simulink model "questao2MiguelSimItem4"  (Simulink 8.7)
settings: Solver=ode45  StartTime=0.0  StopTime=30  MaxStep=0.01  RelTol=1e-3
values from neighbouring files (symbols this model uses):
  A = [0 1  0              0 ... (first row only)    [MatLab4p.m]    (also in MatLab5p.m = [     0        1       0        0; MatLab6p_solucao4.m = [     0        1       0        0; MatLab7p.m = [0 1; -5*sqrt(2) -1]; pplane8.m = [)
  Am = blkdiag(M,M)    [MatLab5p.m]    (also in MatLab6p_solucao4.m; questao2Miguel.m = blkdiag(M); questao2MiguelFinal.m = blkdiag(M))
  Am2 = blkdiag(M)    [questao2Miguel.m]    (also in questao2MiguelFinal.m)
  B = [0; 1/M; 0; -1/(M*L)]    [MatLab4p.m]    (also in MatLab5p.m = [ 0    0; MatLab6p_solucao4.m = [ 0    0; MatLab7p.m = [0 ; 10]; pplane8.m = real(A))
  Bm = blkdiag(N,N)    [MatLab5p.m]    (also in MatLab6p_solucao4.m; questao2Miguel.m = blkdiag(N); questao2MiguelFinal.m = blkdiag(N))
  Bm2 = blkdiag(N)    [questao2Miguel.m]    (also in questao2MiguelFinal.m)
  C = [1 0 0 0]    [MatLab4p.m]    (also in MatLab5p.m = [1 0 0 0; MatLab6p_solucao4.m = [1 0 0 0; MatLab7p.m = [1 0]; pplane8.m = imag(A))
  Dsim = zeros(4,1)    [MatLab4p.m]    (also in MatLab5p.m = zeros(4,2); MatLab6p_solucao4.m = zeros(4,2); questao2Miguel.m; questao2MiguelFinal.m)
  g = 9.81    [MatLab4p.m]    (also in PenduloInvertidoNLinear.m; questao2Miguel.m; questao2MiguelFinal.m)
  K = place(A,B,[-3 -3.05 -3.1 -3.15])    [MatLab4p.m]    (also in MatLab5p.m = Ka(:,1:4); MatLab6p_solucao4.m = Ka(:,1:4); MatLab7p.m = place(A,B,[-4 -4.05]); pplane8.m = kk +2*(jj-1))
  K2 = Ka2(1:4)    [questao2Miguel.m]    (also in questao2MiguelFinal.m)
  Km = Ka(:,5:10)    [MatLab5p.m]    (also in MatLab6p_solucao4.m = Ka(:,5:12); MatLab7p.m = Ka(1,3); questao2Miguel.m = Ka(5); questao2MiguelFinal.m = Ka(5))
  Km2 = Ka2(5:6)    [questao2Miguel.m]    (also in questao2MiguelFinal.m)
  L = (place(A',C',[-9 -9.05 -9.1 -9.15]))'    [MatLab4p.m]    (also in MatLab7p.m = [23 ; 113.9289]; PenduloInvertidoNLinear.m = 1; pplane8.m = length(t); questao2Miguel.m = 1)
  Lobs = H'    [MatLab6p_solucao4.m]    (also in questao2Miguel.m; questao2MiguelFinal.m)
  m = 0.5    [MatLab4p.m]    (also in PenduloInvertidoNLinear.m; questao2Miguel.m; questao2MiguelFinal.m)
  Mcar = 1    [questao2MiguelFinal.m]
  x0 = [0 0 pi/4 0]    [MatLab4p.m]    (also in MatLab5p.m = [1 0.5 1 0.1]; MatLab6p_solucao4.m = [0 0 0 0]; MatLab7p.m = [0 ; 0]; questao2Miguel.m = [0 0.01 0.3 0])
  x0obs = [0 0 0 0]    [MatLab4p.m]    (also in MatLab6p_solucao4.m; MatLab7p.m = [0 ; 0]; questao2Miguel.m; questao2MiguelFinal.m)
settings Model: Creator=hector  LastModifiedBy=Deinis-UFSC
settings DebuggingCC: UnderspecifiedInitializationDetection=Simplified  MergeDetectMultiDrivingBlocksExec=error  SolverPrmCheckMsg=warning
settings ConfigComp: CovSFcnEnable=off

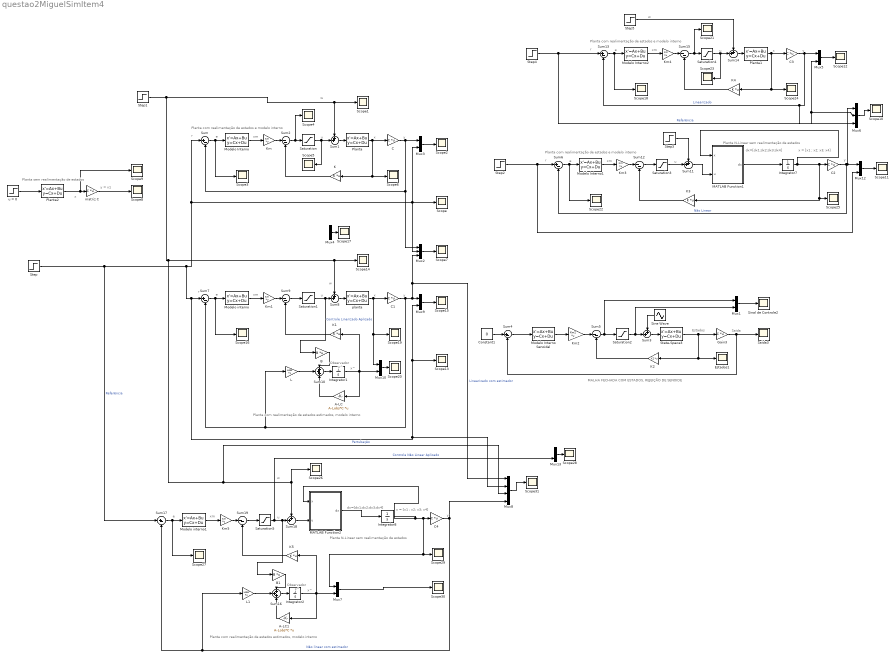
== system questao2MiguelSimItem4 ==
  note: Planta com realimentação de estados estimados, modelo interno
  note: Planta com realimentação de estados e modelo interno
  note: w
  note: u
  note: xm
  note: e
  note: r
  note: x
  note: y
  note: w
  note: u
  note: xm
  note: e
  note: r
  note: x
  note: y
  note: Observador
  note: x^
  note: x^
  note: Planta sem realimentação de estados
  note: x
  note: y = x1
  note: MALHA FECHADA COM ESTADOS, REJEIÇÃO DE SENOIDE
  note: Saida
  note: Estados
  note: Planta com realimentação de estados e modelo interno
  note: u
  note: xm
  note: e
  note: r
  note: y
  note: Planta N-Linear sem realimentação de estados
  note: dx=[dx1;dx2;dx3;dx4]
  note: x = [x1 ; x2; x3; x4]
  note: Planta com realimentação de estados e modelo interno
  note: w
  note: u
  note: xm
  note: e
  note: r
  note: x
  note: y
  note: Planta com realimentação de estados estimados, modelo interno
  note: w
  note: u
  note: xm
  note: e
  note: y
  note: Observador
  note: x^
  note: x^
  note: Planta N-Linear sem realimentação de estados
  note: dx=[dx1;dx2;dx3;dx4]
  note: x = [x1 ; x2; x3; x4]
  A-LC : Gain  Gain=A-Lobs*C  Multiplication=Matrix(K*u)
  A-LC1 : Gain  Gain=A-Lobs*C  Multiplication=Matrix(K*u)
  B : Gain  Gain=B  Multiplication=Matrix(K*u)
  B1 : Gain  Gain=B  Multiplication=Matrix(K*u)
  C{,1..4} (5 alike) : Gain  Gain=C  Multiplication=Matrix(K*u)
  Constant1 : Constant  Value=0
  Estados1 : Scope
  Gain3 : Gain  Gain=C  Multiplication=Matrix(K*u)
  Integrator1 : Integrator  InitialCondition=x0obs
  Integrator2 : Integrator  InitialCondition=x0obs
  Integrator7 : Integrator  InitialCondition=x0
  Integrator8 : Integrator  InitialCondition=x0
  K{,1,3..5} (5 alike) : Gain  Gain=K  Multiplication=Matrix(K*u)
  K2 : Gain  Gain=K2  Multiplication=Matrix(K*u)
  Km{,1,3..5} (5 alike) : Gain  Gain=Km  Multiplication=Matrix(K*u)
  Km2 : Gain  Gain=Km2  Multiplication=Matrix(K*u)
  L : Gain  Gain=Lobs  Multiplication=Matrix(K*u)
  L1 : Gain  Gain=Lobs  Multiplication=Matrix(K*u)
  MATLAB Function1 : MATLAB Function  TreatAsAtomicUnit=on
  MATLAB Function2 : MATLAB Function  TreatAsAtomicUnit=on
  Modelo Interno : StateSpace  A=Am  B=Bm  D=0  X0=0
  Modelo Interno Senoidal : StateSpace  A=Am2  B=Bm2  C=eye(2)  D=zeros(2, 1)  X0=0
  Modelo Interno1 : StateSpace  A=Am  B=Bm  D=0  X0=0
  Modelo Interno2 : StateSpace  A=Am  B=Bm  D=0  X0=0
  Modelo interno : StateSpace  A=Am  B=Bm  D=0  X0=0
  Modelo interno1 : StateSpace  A=Am  B=Bm  D=0  X0=0
  Mux{1,3..5,7,9..10,12..13} (9 alike) : Mux  Inputs=2
  Mux2 : Mux  Inputs=3
  Mux6 : Mux  Inputs=3
  Mux8 : Mux
  Planta : StateSpace  A=A  B=B  C=eye(4)  D=Dsim  X0=x0
  Planta1 : StateSpace  A=A  B=B  C=eye(4)  D=Dsim  X0=x0
  Planta2 : StateSpace  A=A  B=B  C=eye(4)  D=Dsim  X0=x0
  Saida3 : Scope
  Saturation : Saturate  UpperLimit=20  LowerLimit=-20
  Saturation{1..5} (5 alike) : Saturate  UpperLimit=50  LowerLimit=-50
  Scope{,1..31} (32 alike) : Scope
  Sinal de Controle2 : Scope
  Sine Wave : Sin  Amplitude=5  Frequency=0.1  SampleTime=0
  State-Space3 : StateSpace  A=A  B=B  C=eye(4)  D=Dsim  X0=x0
  Step : Step  Time=5  After=0.1  SampleTime=0
  Step1 : Step  Time=15  After=0.5  SampleTime=0
  Step2 : Step  Time=15  After=10  SampleTime=0
  Step3 : Step  Time=30  SampleTime=0
  Step4 : Step  Time=15  After=10  SampleTime=0
  Step5 : Step  Time=30  SampleTime=0
  Sum{,4,6..7,13,17} (6 alike) : Sum  Inputs=|+-
  Sum{1,3,8,11,14,18} (6 alike) : Sum  Inputs=++|
  Sum10 : Sum  Inputs=+++
  Sum{2,5,9,12,15,19} (6 alike) : Sum  Inputs=|--
  Sum16 : Sum  Inputs=+++
  matriz C : Gain  Gain=C  Multiplication=Matrix(K*u)
  planta : StateSpace  A=A  B=B  C=eye(4)  D=Dsim  X0=x0
  "u = 0 " : Step  Time=0  After=0  SampleTime=0
  wires:
  Sum/1 -> Modelo Interno/1, Scope3/1
  Sum1/1 -> Planta/1
  Planta/1 -> C/1, Scope6/1, K/1
  Mux3/1 -> Scope2/1
  Sum2/1 -> Saturation/1, Scope4/1
  Km/1 -> Sum2/1
  Modelo Interno/1 -> Km/1
  K/1 -> Sum2/2
  C/1 -> Mux3/1, Sum/2, Mux2/1
  Saturation/1 -> Sum1/2, Scope5/1
  Sum7/1 -> Modelo interno/1, Scope16/1
  Sum8/1 -> planta/1
  planta/1 -> C1/1, Scope19/1, Mux10/1
  Mux9/1 -> Scope15/1
  Sum9/1 -> Saturation1/1
  Km1/1 -> Sum9/1
  Modelo interno/1 -> Km1/1
  K1/1 -> Sum9/2
  Sum10/1 -> Integrator1/1
  L/1 -> Sum10/2
  A-LC/1 -> Sum10/3
  Integrator1/1 -> Mux10/2, A-LC/1, K1/1
  B/1 -> Sum10/1
  Mux10/1 -> Scope20/1
  Mux2/1 -> Scope7/1
  "u = 0 "/1 -> Planta2/1
  matriz C/1 -> Scope8/1
  Planta2/1 -> Scope9/1, matriz C/1
  State-Space3/1 -> Gain3/1, K2/1, Estados1/1
  Gain3/1 -> Sum4/2, Saida3/1
  Sum4/1 -> Modelo Interno Senoidal/1
  Modelo Interno Senoidal/1 -> Km2/1
  Km2/1 -> Sum5/1
  K2/1 -> Sum5/2
  Sum3/1 -> State-Space3/1
  Sine Wave/1 -> Sum3/1
  Sum5/1 -> Saturation2/1, Mux1/1
  Saturation2/1 -> Sum3/2, Mux1/2
  Mux1/1 -> Sinal de Controle2/1
  Constant1/1 -> Sum4/1
  Mux4/1 -> Scope17/1
  Sum6/1 -> Modelo Interno1/1, Scope22/1
  Mux12/1 -> Scope11/1
  Km3/1 -> Sum12/1
  Modelo Interno1/1 -> Km3/1
  K3/1 -> Sum12/2
  Step3/1 -> Sum11/1
  Sum11/1 -> MATLAB Function1/2(u)
  MATLAB Function1/1(dx) -> Integrator7/1
  C2/1 -> Mux12/1, Mux6/1, Sum6/2  "Não Linear"
  Integrator7/1 -> MATLAB Function1/1(x), K3/1, Scope25/1, C2/1
  Sum12/1 -> Saturation3/1
  Saturation3/1 -> Sum11/2
  Step2/1 -> Mux12/2, Sum6/1
  Sum13/1 -> Modelo Interno2/1, Scope18/1
  Sum14/1 -> Planta1/1
  Planta1/1 -> C3/1, Scope24/1, K4/1
  Mux5/1 -> Scope12/1
  Sum15/1 -> Saturation4/1, Scope21/1
  Km4/1 -> Sum15/1
  Modelo Interno2/1 -> Km4/1
  K4/1 -> Sum15/2
  C3/1 -> Mux5/1, Mux6/3, Sum13/2  "Linearizado"
  Step4/1 -> Mux6/2, Mux5/2, Sum13/1  "Referência"
  Saturation4/1 -> Sum14/2, Scope23/1
  Step5/1 -> Sum14/1
  Mux6/1 -> Scope10/1
  Step/1 -> Sum17/1, Sum/1, Mux2/2, Scope/1, Mux3/2, Sum7/1, Mux8/2, Scope13/1, Mux9/2  "Referência"
  Sum17/1 -> Modelo interno1/1, Scope27/1
  Sum19/1 -> Saturation5/1
  Km5/1 -> Sum19/1
  Modelo interno1/1 -> Km5/1
  K5/1 -> Sum19/2
  Sum16/1 -> Integrator2/1
  L1/1 -> Sum16/2
  A-LC1/1 -> Sum16/3
  B1/1 -> Sum16/1
  Mux7/1 -> Scope30/1
  Mux13/1 -> Scope28/1
  Sum18/1 -> MATLAB Function2/2(u)
  MATLAB Function2/1(dx) -> Integrator8/1
  C4/1 -> Mux8/4, L1/1, Sum17/2  "Não linear com estimador"
  Saturation5/1 -> Mux13/2, B1/1, Sum18/2  "Controle Não Linear Aplicado"
  Integrator2/1 -> A-LC1/1, Mux7/2, K5/1
  Integrator8/1 -> Mux7/1, Scope29/1, C4/1, MATLAB Function2/1(x)
  Mux8/1 -> Scope31/1
  C1/1 -> Mux8/1, Mux2/3, Mux9/1, L/1, Sum7/2  "Linearizado com estimador"
  Step1/1 -> Mux8/3, Sum18/1, Scope26/1, Sum8/1, Scope14/1, Sum1/1, Scope1/1  "Pertubação"
  Saturation1/1 -> B/1, Sum8/2  "Controle Linerizado Aplicado"

== matlab function MATLAB Function1 ==
  data: x input double; u input double; dx output double; m parameter double; Mcar parameter double; L parameter double; g parameter double
function dx = fcn(x,u,m, Mcar, L, g)
%#codegen

% dx1 = x(2);
% dx2 = u - (m*g*cos(x(3))*sin(x(3))+m*L*x(4)^2*sin(x(3)))/(Mcar+m - m*cos(x(3))^2);
% dx3 = x(4);
% dx4 = (u*cos(x(3))+m*L*x(4)^2*cos(x(3))*sin(x(3))-(Mcar+m)*g*sin(x(3)))/(m*L*cos(x(3))^2 - L*(Mcar+m));

dx1 = x(2);
dx2 = (m*L*x(4)^2*sin(x(3))-m*g*sin(x(3))*cos(x(3)) + u)/((Mcar+m*sin(x(3))^2)*L);
dx3 = x(4);
dx4 = ((Mcar+m)*g*sin(x(3)) + m*L*x(4)^2*sin(x(3))*cos(x(3)) - u*cos(x(3)))/((Mcar+m*sin(x(3))^2)*L);

dx = [dx1 ; dx2 ; dx3 ; dx4];

== matlab function MATLAB Function2 ==
  data: x input double; u input double; dx output double; m parameter double; Mcar parameter double; L parameter double; g parameter double
function dx = fcn(x,u,m, Mcar, L, g)
%Miguel 

% dx1 = x(2);
% dx2 = u - (m*g*cos(x(3))*sin(x(3))+m*L*x(4)^2*sin(x(3)))/(Mcar+m - m*cos(x(3))^2);
% dx3 = x(4);
% dx4 = (u*cos(x(3))+m*L*x(4)^2*cos(x(3))*sin(x(3))-(Mcar+m)*g*sin(x(3)))/(m*L*cos(x(3))^2 - L*(Mcar+m));

dx1 = x(2);
dx2 = (m*L*x(4)^2*sin(x(3))-m*g*sin(x(3))*cos(x(3)) + u)/((Mcar+m*sin(x(3))^2)*L);
dx3 = x(4);
dx4 = ((Mcar+m)*g*sin(x(3)) + m*L*x(4)^2*sin(x(3))*cos(x(3)) - u*cos(x(3)))/((Mcar+m*sin(x(3))^2)*L);


dx = [dx1 ; dx2 ; dx3 ; dx4];
